simulink model "model_response"  (R2024b)
settings: Solver=VariableStepAuto  StartTime=0.0  StopTime=10  RelTol=1e-3
values from neighbouring files (symbols this model uses):
  A = [-1.48429 1 0 0 -70.19827 0 1 0 -62.7051681 0 0 1 ... (16 elements, 4x4)]    [state_space.mat]    (also in problem2.m = SS.A; problem2_sub.m = SS.A'; problem3.m = SS.A; problem4.m = SS.A)
  B = [1 0 0 0]    [state_space.mat]    (also in problem2.m = SS.B; problem2_sub.m = SS.C'; problem3.m = SS.B; problem4.m = SS.B)
  C = [0 0.177827941004 0.0245455906968 3.76447542653]    [state_space.mat]    (also in problem2.m = SS.C; problem2_sub.m = SS.B'; problem3.m = SS.C; problem4.m = SS.C)
  F = pinv(C * (Acl \ B))    [problem2.m]    (also in problem3.m = Cl.F; problem4.m = SVF.F; problen2_thomas.m = inv(C * inv(-A + B*K) * B))
  K = place(A,B,Desired_poles)    [problem2.m]    (also in problem3.m = Cl.K; problem4.m = SVF.K; problen2_thomas.m)
  u_amp = 1    [problem3.m]    (also in problem5.m = 0.169102975876)
  u_w = 2 * pi    (= 6.28318530718)    [problem3.m]    (also in problem5.m)
  useSine = true    [problem3.m]    (also in problem5.m)
settings Model: Creator=carso  LastModifiedBy=owencraig

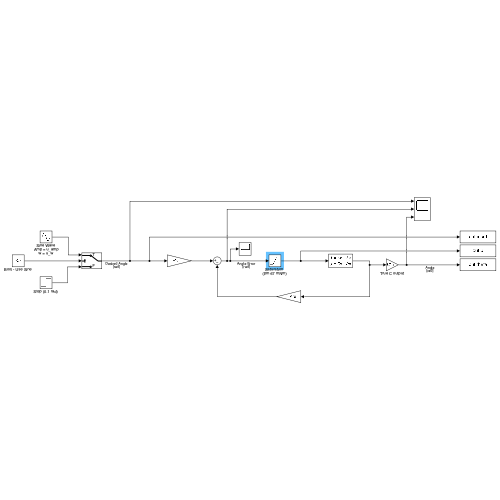
[thumbnail: Simulink's stored preview of the top-level diagram]
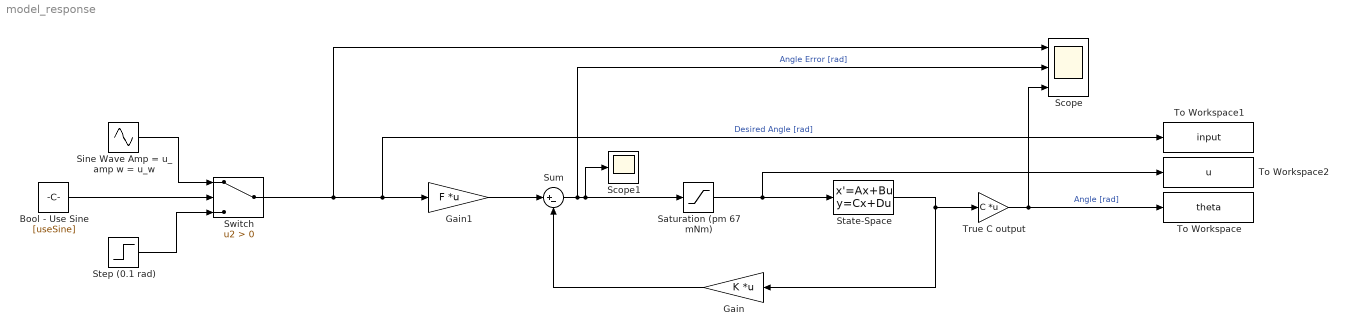
== system model_response ==
  Bool - Use Sine : Constant  Value=[useSine]
  Gain : Gain  Gain=K  Multiplication=Matrix(K*u)
  Gain1 : Gain  Gain=F  Multiplication=Matrix(K*u)
  Saturation (pm 67 mNm) : Saturate  UpperLimit=67  LowerLimit=-67
  Scope : Scope  NumInputPorts=3
  Scope1 : Scope
  Sine Wave Amp = u_amp w = u_w : Sin  Amplitude=[u_amp]  Frequency=[u_w]  SampleTime=0
  State-Space : StateSpace  A=A  B=B  C=eye(4)  D=zeros(4,1)  InitialCondition=0
  Step (0.1 rad) : Step  After=0.1  SampleTime=0
  Sum : Sum  Inputs=|+-
  Switch : Switch  Criteria=u2 > Threshold  SaturateOnIntegerOverflow=off  InputSameDT=off
  To Workspace : ToWorkspace  VariableName=theta  SaveFormat=Timeseries  SampleTime=-1
  To Workspace1 : ToWorkspace  VariableName=input  SaveFormat=Timeseries  SampleTime=-1
  To Workspace2 : ToWorkspace  VariableName=u  SaveFormat=Timeseries  SampleTime=-1
  True C output : Gain  Gain=C  Multiplication=Matrix(K*u)
  wires:
  Sum/1 -> Scope/2, Scope1/1, Saturation (pm 67 mNm)/1  "Angle Error [rad]"
  True C output/1 -> To Workspace/1, Scope/3  "Angle [rad]"
  Switch/1 -> Scope/1, To Workspace1/1, Gain1/1  "Desired Angle [rad]"
  Bool - Use Sine/1 -> Switch/2
  Step (0.1 rad)/1 -> Switch/3
  Sine Wave Amp = u_amp w = u_w/1 -> Switch/1
  Saturation (pm 67 mNm)/1 -> To Workspace2/1, State-Space/1
  Gain/1 -> Sum/2
  State-Space/1 -> True C output/1, Gain/1
  Gain1/1 -> Sum/1
